simulink model "tp1_simulink_d"  (R2024a)
settings: Solver=VariableStepAuto  StartTime=0.0  StopTime=10.0  RelTol=1e-3
libraries: cstblocks x2
settings Model: Creator=tiago  LastModifiedBy=tiago

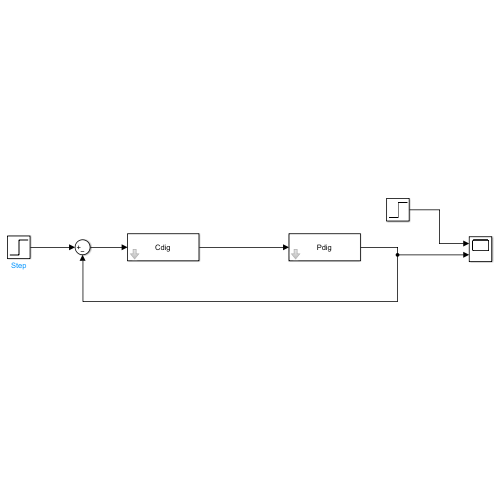
[thumbnail: Simulink's stored preview of the top-level diagram]
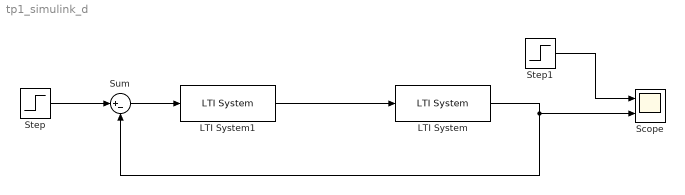
== system tp1_simulink_d ==
  LTI System : cstblocks/LTI System  sys=Pdig  IC=[]  PadeOrder=0
  LTI System1 : cstblocks/LTI System  sys=Cdig  IC=[]  PadeOrder=0
  Scope : Scope  NumInputPorts=2
  Step : Step  SampleTime=0
  Step1 : Step  SampleTime=0
  Sum : Sum  Inputs=|+-
  wires:
  Sum/1 -> LTI System1/1
  LTI System1/1 -> LTI System/1
  Step/1 -> Sum/1
  LTI System/1 -> Scope/2, Sum/2
  Step1/1 -> Scope/1
